simulink model "Ejercicio_3_b"  (R2023a)
settings: Solver=VariableStepAuto  StartTime=0.0  StopTime=5  RelTol=1e-3
values from neighbouring files (symbols this model uses):
  g0 = utilsMati.realim_VE.factorEscala(A,B,C,K)    [Resolucion.m]
  K = acker(A, B, PLC_VE)    [Resolucion.m]
  Ke = acker(A',C',PLC_VE)'    [Resolucion.m]
undefined symbols (not defined in the file or in its folder): A, B, C
settings Model: Creator=Mati  LastModifiedBy=Mati

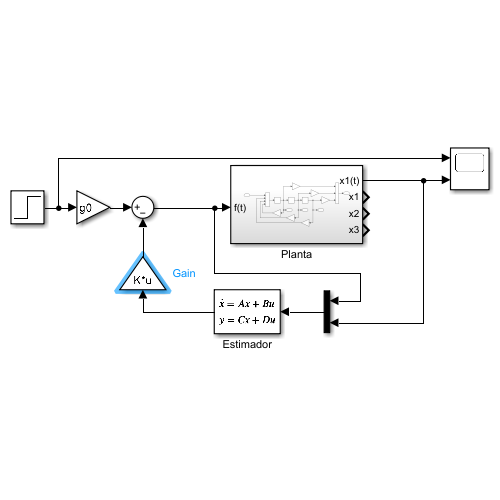
[thumbnail: Simulink's stored preview of the top-level diagram]
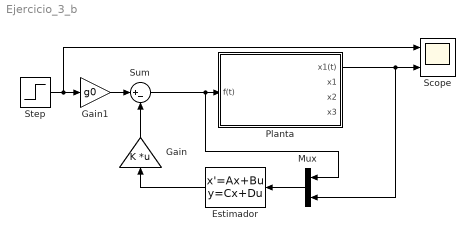
== system Ejercicio_3_b ==
  Estimador : StateSpace  A=A-Ke*C  B=[B Ke]  C=eye(3)  D=[0 0 0; 0 0 0]'  InitialCondition=0
  Gain : Gain  Gain=K  Multiplication=Matrix(K*u)
  Gain1 : Gain  Gain=g0
  Mux : Mux  Inputs=2
  Planta : Subsystem
  Scope : Scope  NumInputPorts=2
  Step : Step  SampleTime=0
  Sum : Sum  Inputs=|+-
  wires:
  Step/1 -> Scope/1, Gain1/1
  Gain1/1 -> Sum/1
  Sum/1 -> Mux/1, Planta/1(f(t))
  Gain/1 -> Sum/2
  Estimador/1 -> Gain/1
  Mux/1 -> Estimador/1
  Planta/1(x1(t)) -> Mux/2, Scope/2

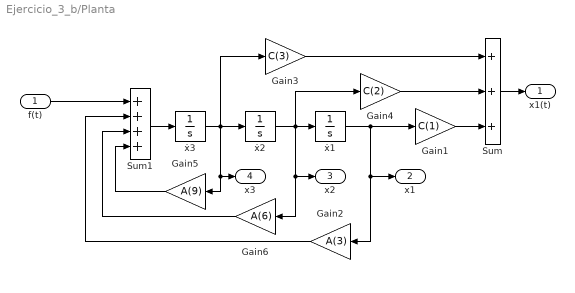
== system Ejercicio_3_b/Planta ==
  f(t) : Inport
  Gain1 : Gain  Gain=C(1)
  Gain2 : Gain  Gain=A(3)
  Gain3 : Gain  Gain=C(3)
  Gain4 : Gain  Gain=C(2)
  Gain5 : Gain  Gain=A(9)
  Gain6 : Gain  Gain=A(6)
  Sum : Sum  Inputs=+++
  Sum1 : Sum  Inputs=++++
  ẋ1 : Integrator
  ẋ2 : Integrator
  ẋ3 : Integrator
  x1(t) : Outport
  x1 : Outport  Port=2
  x2 : Outport  Port=3
  x3 : Outport  Port=4
  wires:
  f(t)/1 -> Sum1/1
  Sum1/1 -> ẋ3/1
  ẋ3/1 -> x3/1, Gain5/1, Gain3/1, ẋ2/1
  ẋ2/1 -> x2/1, Gain6/1, Gain4/1, ẋ1/1
  ẋ1/1 -> x1/1, Gain2/1, Gain1/1
  Sum/1 -> x1(t)/1
  Gain5/1 -> Sum1/4
  Gain6/1 -> Sum1/3
  Gain2/1 -> Sum1/2
  Gain1/1 -> Sum/3
  Gain4/1 -> Sum/2
  Gain3/1 -> Sum/1
